simulink model "sm_cart_double_pendulum"  (R2021b)
settings: Solver=ode45  StartTime=0.0  StopTime=10  MaxStep=0.01  RelTol=1e-6  AbsTol=1e-6  EnableMultiTasking=on
undefined symbols (not defined in the file): sys_cart_dpen, X, Y, Z
libraries: sm_lib x23, nesl_utility x9, simulink x1
CloseFcn:
  | clear sys_cart_dpen
Description:
  | Inverted Double Pendulum on a Sliding Cart
  | 
  | This example shows how to model an inverted double pendulum mounted on a sliding cart using Simscape Multibody(TM). It also illustrates the use of a controller to balance the pendulum in the upright position. Make any changes to the system and click on the blue box to generate linearized model for the system before running the simulation. The control gains are computed using the linearized model. The pole placement technique is used to compute the control gains from the linearized model. The controller keeps the double pendulum vertical in the presence of a random disturbance force. See the files sm_cart_dpen_linearize.m and sm_cart_dpen_control_gains.m for details.
settings Model: Creator=The MathWorks, Inc.  LastModifiedBy=The MathWorks, Inc.
settings SolverCC: AutoScaleAbsTol=off  AlgebraicLoopSolver=TrustRegion
settings DataIOCC: LimitDataPoints=on  SaveFormat=Array  SaveOutput=off  SignalLogging=off  SaveTime=off  ReturnWorkspaceOutputs=off
settings OptimizationCC: DefaultParameterBehavior=Inlined  BufferReuse=off  ExpressionDepthLimit=2147483647  LifeSpan=inf
settings DebuggingCC: UnderspecifiedInitializationDetection=Classic  MergeDetectMultiDrivingBlocksExec=none  SolverPrmCheckMsg=warning  FcnCallInpInsideContextMsg=warning  UnconnectedInputMsg=none  AllowSymbolicDim=off  StateNameClashWarn=warning  InitInArrayFormatMsg=none  SFUnexpectedBacktrackingDiag=warning  SFNoUnconditionalDefaultTransitionDiag=warning  SFExecutionAtInitializationDiag=none  SFMachineParentedDataDiag=warning  ArithmeticOperatorsInVariantConditions=warning
settings HardwareCC: ProdBitPerPointer=32  ProdBitPerSizeT=32  ProdBitPerPtrDiffT=32  ProdLargestAtomicFloat=None  ProdIntDivRoundTo=Undefined  ProdEndianess=Unspecified  ProdWordSize=32  ProdHWDeviceType=32-bit Generic
settings ModelReferenceCC: PropagateSignalLabelsOutOfModel=off
settings SFSimCC: SimUseLocalCustomCode=off  CustomCodeUndefinedFunction=UseInterfaceOnly
settings RTWCC: RTWUseLocalCustomCode=off
settings CodeAppCC: StateflowObjectComments=on
settings GRTTargetCC: TargetLangStandard=C89/C90 (ANSI)  CombineOutputUpdateFcns=off  GRTInterface=on
settings ConfigComp: CovMetricSettings=dw  CovSaveCumulativeToWorkspaceVar=on  CovSaveSingleToWorkspaceVar=on  CovExternalEMLEnable=off  CovSFcnEnable=off
settings SimscapeCC: SimscapeNormalizeSystem=off
settings ConfigurationSet: Description=SimMechanics 2G
settings ExplorerConfigSet: InternalSimMechanicsExplorerSettings="<ExplorerConfiguration><canonicalview>default</canonicalview><TilePanel><TileInfo><Tiles Columns=\"1\" Count=\"1\" Rows=\"1\"><Column Left=\"2\" Weight=\"1\"/><Column Left=\"461\"/><Row Top=\"2\" Weight=\"1\"/><Row Top=\"419\"/><Tile Height=\"1\" Width=\"1\" X=\"0\" Y=\"0\"/></Tiles></TileInfo><SceneInfo><SceneViewer><BGColor><R>0.60000002384185791</R><G>0.60000002384185791</G><B>0.60000002384185791</B></BGColor><Camera><Position><X>0.59825210896441083</X><Y>-0.62075210985848051</Y><Z>0.77498517063566785</Z></Position><Center><X>0</X><Y>-0.022500000894069672</Y><Z>0.17673306167125702</Z></Center><Up><X>-0.40824829046386307</X><Y>0.40824829046386307</Y><Z>0.81649658092772615</Z></Up><Left>-0.2914164036512375</Left><Right>0.2914164036512375</Right><Bottom>-0.31976635158061983</Bottom><Top>0.31976635158061983</Top></Camera></SceneViewer></SceneInfo></TilePanel></ExplorerConfiguration>"

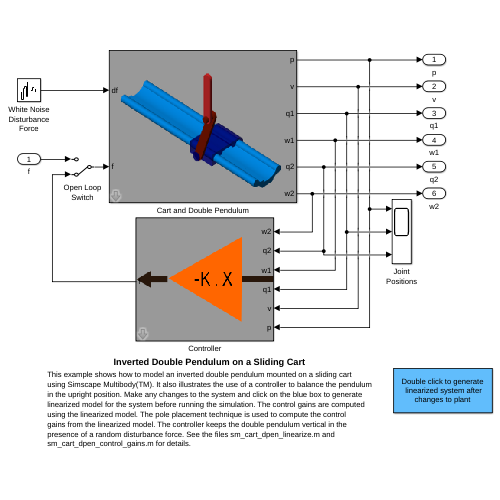
[thumbnail: Simulink's stored preview of the top-level diagram]
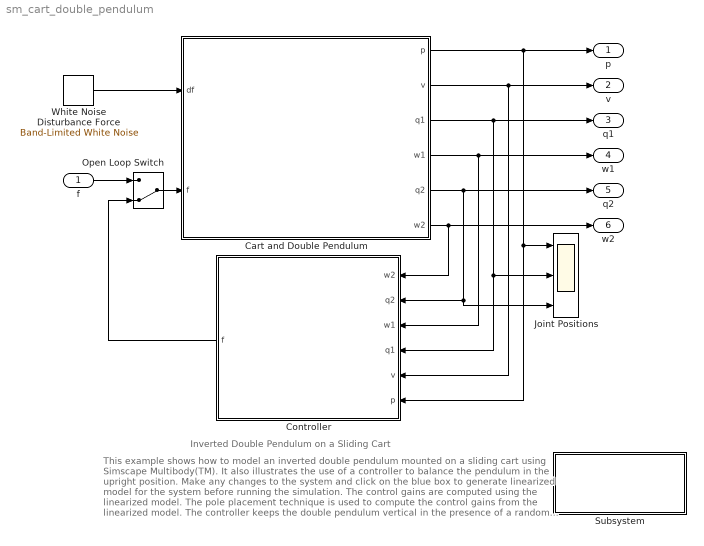
== system sm_cart_double_pendulum ==
  note: This example shows how to model an inverted double pendulum mounted on a sliding cart
      | using Simscape Multibody(TM). It also illustrates the use of a controller to balance the pendulum
      | in the upright position. Make any changes to the system and click on the blue box to generate
      | linearized model for the system before running the simulation. The control gains are computed
      | using the linearized model. The pole placement technique is used to compute the control
      | gains from the linearized model. The controller keeps the double pendulum vertical in the
      | presence of a random disturbance force. See the files sm_cart_dpen_linearize.m and
      | sm_cart_dpen_control_gains.m for details.
  note: Inverted Double Pendulum on a Sliding Cart
  f : Inport
  Cart and Double Pendulum : Subsystem  mask(Double Pendulum on a Sliding Cart){Ll=18, Lu=14, p=7, v=0, q1=-20, w1=0, q2=20, w2=0}
      mask prompts: Ll "Lower link length (cm)"; Lu "Upper link length (cm)"; p "Cart initial position (cm)"; v "Cart initial velocity (cm/s)"; q1 "Lower link initial position (deg)"; w1 "Lower link initial velocity (deg/s)"; q2 "Upper link initial position (deg)"; w2 "Upper link initial velocity (deg/s)"
      mask help:
      | Set the lengths of the pendulum links and the initial states of the joint positions and velocities in the dialog below. For other changes to the system, right click on the block and select Look Under Mask to edit the system directly.
      |
      | After any changes to the system, double click on the blue box titled "Double click to linearize system" before proceeding to simulate the model. This generates the linearized model (about the vertical upright position) of the system. The linearized system is used by the controller to compute the control gains.
      mask Display:
      | image('sm_cartdpen_full.png');
      | port_label('input',1,'df');
      | port_label('input',2,'f');
      | port_label('output',1,'p');
      | port_label('output',2,'v');
      | port_label('output',3,'q1');
      | port_label('output',4,'w1');
      | port_label('output',5,'q2');
      | port_label('output',6,'w2');
  Controller : Subsystem  mask(Controller){poles=[-11 -10 -10 -10 -10 -10], sys=sys_cart_dpen}
      mask prompts: poles "Closed Loop Desired Pole Locations (1x6 vector)"; sys "Linearized system model"
      mask help: The controller gains are computed using the Ackermann's formula for pole placement. Specify the desired closed loop pole locations (1x6 vector) in the dialog below.
      mask init:
      | if isempty(sys)
      |     K_pp = [70.5210   41.6715 -110.3868  -24.2497 -218.6747  -18.6261];
      |     Cinv = diag([1/100 1/100 1/57.2958 1/57.2958 1/57.2958 1/57.2958]);
      | else
      |     K_pp = sm_cart_dpen_control_gains(sys,poles);
      |     Cinv = inv(sys.C);
      | end
      mask Display:
      | image('sm_cartdpen_ctrl.png');
      | port_label('output',1,'f');
      | port_label('input',6,'p');
      | port_label('input',5,'v');
      | port_label('input',4,'q1');
      | port_label('input',3,'w1');
      | port_label('input',2,'q2');
      | port_label('input',1,'w2');
  Joint Positions : Scope  NumInputPorts=3
  Open Loop Switch : ManualSwitch  CurrentSetting=0
  Subsystem : Subsystem
      settings: OpenFcn=sm_cart_dpen_linearize();
      mask Display: disp('Double click to generate\n linearized system after\nchanges to plant');
  White Noise Disturbance Force : simulink/Sources/Band-Limited White Noise  Cov=1e-4  Ts=0.1  seed=[23341]
  p : Outport  VectorParamsAs1DForOutWhenUnconnected=off
  v : Outport  Port=2  VectorParamsAs1DForOutWhenUnconnected=off
  q1 : Outport  Port=3  VectorParamsAs1DForOutWhenUnconnected=off
  w1 : Outport  Port=4  VectorParamsAs1DForOutWhenUnconnected=off
  q2 : Outport  Port=5  VectorParamsAs1DForOutWhenUnconnected=off
  w2 : Outport  Port=6  VectorParamsAs1DForOutWhenUnconnected=off
  wires:
  f/1 -> Open Loop Switch/1
  Open Loop Switch/1 -> Cart and Double Pendulum/2(f)
  Cart and Double Pendulum/6(w2) -> Controller/1(w2), w2/1
  Cart and Double Pendulum/5(q2) -> q2/1, Joint Positions/3, Controller/2(q2)
  Cart and Double Pendulum/4(w1) -> Controller/3(w1), w1/1
  Cart and Double Pendulum/3(q1) -> q1/1, Controller/4(q1), Joint Positions/2
  Cart and Double Pendulum/2(v) -> Controller/5(v), v/1
  Cart and Double Pendulum/1(p) -> p/1, Controller/6(p), Joint Positions/1
  Controller/1(f) -> Open Loop Switch/2
  White Noise Disturbance Force/1 -> Cart and Double Pendulum/1(df)

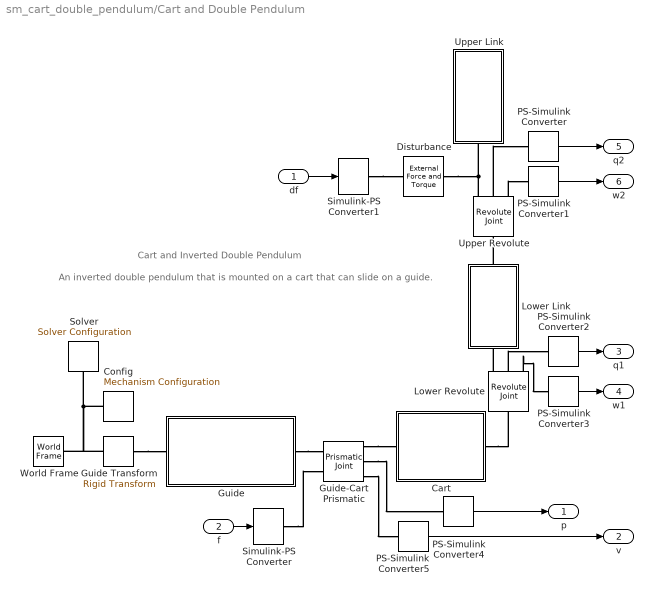
== system sm_cart_double_pendulum/Cart and Double Pendulum ==
  note: An inverted double pendulum that is mounted on a cart that can slide on a guide.
  note: Cart and Inverted Double Pendulum
  df : Inport
  f : Inport  Port=2
  Cart : Subsystem  mask(Cart){W=10, Rs=1.2, Rm=2, L=10, Rp=1, Lp=2, Rf=1.5, Tf=0.25, rho=2700, Op=0.6}
      mask prompts: W "Cart width (cm)"; Rs "Slider cavity radius (cm)"; Rm "Radius of curvature of outer surface (cm)"; L "Cart length (cm)"; Rp "Peg radius (cm)"; Lp "Peg length (cm)"; Rf "Peg Flange radius (cm)"; Tf "Peg flange thickness (cm)"; rho "Density"; Op "Opacity (cm)"
      mask help: Cart slides on a guide structure and has a peg to hang the double pendulum
      mask init:
      | theta = (180:-1:-90)*pi/180;
      | cx = W/2; cy = 0;
      | x1 = cx + 1.1*Rs*cos(theta');
      | y1 = cy + 1.1*Rs*sin(theta');
      | 
      | theta = (-90:1:90)*pi/180;
      | cx = W/2; cy = 0;
      | x2 = cx + Rm*cos(theta');
      | y2 = cy + Rm*sin(theta');
      | 
      | x3 = [-(W/2+Rm); -(W/2+Rm); -W/2];
      | y3 = [Rm; -Rm; -Rm];
      | 
      | x = [x1; x2; x3];
      | y = [y1; y2; y3];
      | 
      | x = [x ; -flipud(x1); -W/4; -W/5; W/5; W/4];
      | y = [y ;  flipud(y1); 0; Rm/2; Rm/2; 0];
      | 
      | cross_section = [x y];
      mask Display: image('sm_cartdpen_cart.png')
  Config : sm_lib/Utilities/Mechanism Configuration  UniformGravity=Constant  GravityVector=[0 0 -9.81]  GravityUnits=m/s^2  LinearizationDelta=0.001  JointModeTransitionNonlinearIterations=2
  Disturbance : sm_lib/Forces and Torques/External Force and Torque  ForceResolutionFrame=World  EnableForceX=on  EnableForceY=off  EnableForceZ=off  EnableForce=off  TorqueResolutionFrame=AttachedFrame  EnableTorqueX=off  EnableTorqueY=off  EnableTorqueZ=off  EnableTorque=off
  Guide : Subsystem  mask(Guide){W=10, Rs=1.2, Rm=3, Rl=6, L=60, Rg=1.5, rho=2700}
      mask prompts: W "Guide width (cm)"; Rs "Slider rod radius (cm)"; Rm "Underside curvature radius (cm)"; Rl "Upperside curvature radius (cm)"; L "Guide length (cm)"; Rg "Center to rack distance (cm)"; rho "Density"
      mask help: Guide structure on which the card slides
      mask init:
      | phi = asin((W/2-Rs)/Rl);
      | theta = (-phi*3/4:(-1/180):-phi) - pi/2;
      | cx = 0; cy = Rm-Rm*sin(25*pi/180)  + Rl*cos(phi) + Rs;
      | 
      | x2 = cx + Rl*cos(theta');
      | y2 = cy + Rl*sin(theta');
      | 
      | theta = (phi:(-1/180):0.01) - pi/2;
      | x5 = cx + Rl*cos(theta');
      | y5 = cy + Rl*sin(theta');
      | 
      | x1 = [0; -Rg; -Rg];
      | y1 = [cy-Rl; cy-Rl; y2(1)];
      | 
      | theta = (0:1:270)*pi/180;
      | cx = -W/2; cy = Rm-Rm*sin(25*pi/180)+Rs;
      | 
      | x3 = cx + Rs*cos(theta');
      | y3 = cy + Rs*sin(theta');
      | 
      | theta = (89:-1:25)*pi/180;
      | cx = -W/2; cy = -Rm*sin(25*pi/180);
      | 
      | x4 = cx + Rm*cos(theta');
      | y4 = cy + Rm*sin(theta');
      | 
      | x = [x1; x2; x3; x4; -flipud([x3;x4]); x5];
      | y = [y1; y2; y3; y4;  flipud([y3;y4]); y5];
      | 
      | cross_section = [x y];
      mask Display: image('sm_cartdpen_guide.png')
  Guide Transform : sm_lib/Frames and Transforms/Rigid Transform  TranslationMethod=None  TranslationStandardOffset=0  TranslationLengthUnit=m  TranslationStandardAxis=+Z  TranslationCartesianOffset=[0 0 0]  TranslationROffset=0  TranslationROffsetUnits=m  TranslationZOffset=0  TranslationZOffsetUnits=m  TranslationThetaOffset=0  TranslationThetaOffsetUnits=deg  RotationMethod=AlignedAxes  RotationAngleUnits=deg  RotationStandardAxis=+Z  RotationAngle=0  RotationArbitraryAxis=[0 0 1]  FollAlignAxisA=+Z  BaseAlignAxisA=+X  FollAlignAxisB=+X  BaseAlignAxisB=+Y  RotationSequenceAxes=FollowerAxes  RotationSequence=XYX  RotationSequenceAngles=[0 0 0]  RotationSequenceAnglesUnits=deg  RotationMatrix=[1 0 0; 0 1 0; 0 0 1]
  Guide-Cart Prismatic : sm_lib/Joints/Prismatic Joint  JointMode=Normal  SenseConstraintForce=off  SenseConstraintForceX=off  SenseConstraintForceY=off  SenseConstraintForceZ=off  SenseConstraintTorque=off  SenseConstraintTorqueX=off  SenseConstraintTorqueY=off  SenseConstraintTorqueZ=off  SenseTotalForce=off  SenseTotalForceX=off  SenseTotalForceY=off  SenseTotalForceZ=off  SenseTotalTorque=off  SenseTotalTorqueX=off  SenseTotalTorqueY=off  SenseTotalTorqueZ=off  CompositeWrenchDir=FollowerOnBase  CompositeWrenchFrame=BaseFrame  EquilibriumPosition=0  EquilibriumPositionUnits=m  SpringStiffness=0  SpringStiffnessUnits=N/m  DampingCoefficient=0  DampingCoefficientUnits=N/(m/s)  TorqueActuationMode=InputTorque  MotionActuationMode=ComputedMotion  SensePosition=on  SenseVelocity=on  SenseAcceleration=off  SenseTorqueForce=off  SenseLowerLimitTorqueForce=off  SenseUpperLimitTorqueForce=off  LowerLimitSpecify=off  LowerLimitBound=-1  LowerLimitBoundUnits=m  LowerLimitStiffness=1e6  LowerLimitStiffnessUnits=N/m  LowerLimitDamping=1e3  LowerLimitDampingUnits=N/(m/s)  LowerLimitTransitionRegionWidth=1e-4  LowerLimitTransitionRegionWidthUnits=m  UpperLimitSpecify=off  UpperLimitBound=1  UpperLimitBoundUnits=m  UpperLimitStiffness=1e6  UpperLimitStiffnessUnits=N/m  UpperLimitDamping=1e3  UpperLimitDampingUnits=N/(m/s)  UpperLimitTransitionRegionWidth=1e-4  UpperLimitTransitionRegionWidthUnits=m  PositionTargetSpecify=on  PositionTargetPriority=High  PositionTargetValue=p  PositionTargetValueUnits=cm  VelocityTargetSpecify=on  VelocityTargetPriority=High  VelocityTargetValue=v  VelocityTargetValueUnits=cm/s
  Lower Link : Subsystem  mask(Upper Link){rho=2700, L=Ll, W=3, T=1, r=1, Lp=3, clr=[0.6 0.1 0]}
      mask prompts: rho "Link density (kg/m^3):"; L "Link length (cm):"; W "Link width (cm):"; T "Link thickness (cm):"; r "Peg/Hole radius (cm):"; Lp "Peg length (cm):"; clr "Link color:"
      mask help: Upper link of the double pendulum mechanisn
      mask init:
      | % Main link cross-section
      | top_xsec = [L/2 W/2; -L/2 W/2];
      | theta = (90:-1:-90)*pi/180;
      | semi_hole_xsec = [-L/2+r*cos(theta') r*sin(theta')];
      | bottom_xsec = [-L/2 -W/2; L/2 -W/2];
      | theta = (-89:1:89)*pi/180;
      | right_end_xsec = [L/2+(W/2)*cos(theta') (W/2)*sin(theta')];
      | link_x_section = [ top_xsec; semi_hole_xsec; bottom_xsec; right_end_xsec];
      | 
      | % Left end cap cross-section
      | theta = (90:1:270)*pi/180;
      | outer_xsec = [(W/2)*cos(theta') (W/2)*sin(theta')];
      | theta = (270:-1:90)*pi/180;
      | inner_xsec = [r*cos(theta') r*sin(theta')];
      | left_end_x_section = [outer_xsec; inner_xsec];
      mask Display: image('sm_cartdpen_lowerlink.png');
  Lower Revolute : sm_lib/Joints/Revolute Joint  JointMode=Normal  SenseConstraintForce=off  SenseConstraintForceX=off  SenseConstraintForceY=off  SenseConstraintForceZ=off  SenseConstraintTorque=off  SenseConstraintTorqueX=off  SenseConstraintTorqueY=off  SenseConstraintTorqueZ=off  SenseTotalForce=off  SenseTotalForceX=off  SenseTotalForceY=off  SenseTotalForceZ=off  SenseTotalTorque=off  SenseTotalTorqueX=off  SenseTotalTorqueY=off  SenseTotalTorqueZ=off  CompositeWrenchDir=FollowerOnBase  CompositeWrenchFrame=BaseFrame  EquilibriumPosition=0  EquilibriumPositionUnits=rad  SpringStiffness=0  SpringStiffnessUnits=N*m/rad  DampingCoefficient=0  DampingCoefficientUnits=N*m/(rad/s)  TorqueActuationMode=NoTorque  MotionActuationMode=ComputedMotion  SensePosition=on  SenseVelocity=on  SenseAcceleration=off  SenseTorqueForce=off  SenseLowerLimitTorqueForce=off  SenseUpperLimitTorqueForce=off  LowerLimitSpecify=off  LowerLimitBound=-90  LowerLimitBoundUnits=deg  LowerLimitStiffness=1e4  LowerLimitStiffnessUnits=N*m/deg  LowerLimitDamping=10  LowerLimitDampingUnits=N*m/(deg/s)  LowerLimitTransitionRegionWidth=0.1  LowerLimitTransitionRegionWidthUnits=deg  UpperLimitSpecify=off  UpperLimitBound=90  UpperLimitBoundUnits=deg  UpperLimitStiffness=1e4  UpperLimitStiffnessUnits=N*m/deg  UpperLimitDamping=10  UpperLimitDampingUnits=N*m/(deg/s)  UpperLimitTransitionRegionWidth=0.1  UpperLimitTransitionRegionWidthUnits=deg  PositionTargetSpecify=on  PositionTargetPriority=High  PositionTargetValue=q1  PositionTargetValueUnits=deg  VelocityTargetSpecify=on  VelocityTargetPriority=Low  VelocityTargetValue=w1  VelocityTargetValueUnits=deg/s
  PS-Simulink Converter : nesl_utility/PS-Simulink Converter  PhysicalDomain=network_engine_domain  SubClassName=ps_output  LeftPortType=input  RightPortType=output  PseudoPeriodic=off  Frequencies=[]  Unit=deg  AffineConversion=off
      settings: SourceProductBaseCode=PW,SS
  PS-Simulink Converter1 : nesl_utility/PS-Simulink Converter  PhysicalDomain=network_engine_domain  SubClassName=ps_output  LeftPortType=input  RightPortType=output  PseudoPeriodic=off  Frequencies=[]  Unit=deg/s  AffineConversion=off
      settings: SourceProductBaseCode=PW,SS
  PS-Simulink Converter2 : nesl_utility/PS-Simulink Converter  PhysicalDomain=network_engine_domain  SubClassName=ps_output  LeftPortType=input  RightPortType=output  PseudoPeriodic=off  Frequencies=[]  Unit=deg  AffineConversion=off
      settings: SourceProductBaseCode=PW,SS
  PS-Simulink Converter3 : nesl_utility/PS-Simulink Converter  PhysicalDomain=network_engine_domain  SubClassName=ps_output  LeftPortType=input  RightPortType=output  PseudoPeriodic=off  Frequencies=[]  Unit=deg/s  AffineConversion=off
      settings: SourceProductBaseCode=PW,SS
  PS-Simulink Converter4 : nesl_utility/PS-Simulink Converter  PhysicalDomain=network_engine_domain  SubClassName=ps_output  LeftPortType=input  RightPortType=output  PseudoPeriodic=off  Frequencies=[]  Unit=cm  AffineConversion=off
      settings: SourceProductBaseCode=PW,SS
  PS-Simulink Converter5 : nesl_utility/PS-Simulink Converter  PhysicalDomain=network_engine_domain  SubClassName=ps_output  LeftPortType=input  RightPortType=output  PseudoPeriodic=off  Frequencies=[]  Unit=cm/s  AffineConversion=off
      settings: SourceProductBaseCode=PW,SS
  Simulink-PS Converter : nesl_utility/Simulink-PS Converter  PhysicalDomain=network_engine_domain  SubClassName=ps_input  LeftPortType=input  RightPortType=output  PseudoPeriodic=off  Frequencies=[]  NoiseDistribution=none  NoiseParameters=[]  Unit=N  AffineConversion=off  FilteringAndDerivatives=zero  SimscapeFilterOrder=1  InputFilterTimeConstant=.001  UdotUserProvided=1
      settings: SourceProductBaseCode=PW,SS
  Simulink-PS Converter1 : nesl_utility/Simulink-PS Converter  PhysicalDomain=network_engine_domain  SubClassName=ps_input  LeftPortType=input  RightPortType=output  PseudoPeriodic=off  Frequencies=[]  NoiseDistribution=none  NoiseParameters=[]  Unit=N  AffineConversion=off  FilteringAndDerivatives=zero  SimscapeFilterOrder=1  InputFilterTimeConstant=.001  UdotUserProvided=1
      settings: SourceProductBaseCode=PW,SS
  Solver : nesl_utility/Solver Configuration  PhysicalDomain=network_engine_domain  SubClassName=solver  LeftPortType=input  RightPortType=generic  Tones=[]  Harmonics=[]  SimulateNoise=off  Profile=off  UseLocalSampling=off  EnableSwitchedLinearOptims=on  FrequencyDomain=off  UseCCode=off  RelTol=0.001  AbsTol=1e-06  MinStep=1e-09  ToWorkspace=off  RevertToSquareIcSolve=off  NumHomotopyIterations=100  PhasorMode=off  PhasorModeNumHarmonics=1  DoDC=off  ResidualTolerance=1e-9  UseLocalSolver=off  LocalSolverChoice=NE_BACKWARD_EULER_ADVANCER  LocalSolverSampleTime=.001  DoFixedCost=off  MaxNonlinIter=3  MaxModeIter=2  ComputeImpulses=off  ImpulseIterations=2  LinearAlgebra=Sparse  EquationFormulation=NE_TIME_EF  DelaysMemoryBudget=1024  AutomaticFiltering=on  FilteringTimeConstant=0.001  PartitionStorageMethod=AS_NEEDED  PartitionMemoryBudget=1024  PartitionMethod=FAST
      settings: SourceProductBaseCode=PW,SS
  Upper Link : Subsystem  mask(Upper Link){rho=2700, L=Lu, W=3, T=1, r=1, clr=[1 0.2 0.2]}
      mask prompts: rho "Link density (kg/m^3):"; L "Link length (cm):"; W "Link width (cm):"; T "Link thickness (cm):"; r "Hole radius (cm):"; clr "Link color:"
      mask help: Upper link of the double pendulum mechanisn
      mask init:
      | % Main link cross-section
      | top_xsec = [L/2 W/2; -L/2 W/2];
      | theta = (90:-1:-90)*pi/180;
      | semi_hole_xsec = [-L/2+r*cos(theta') r*sin(theta')];
      | bottom_xsec = [-L/2 -W/2; L/2 -W/2];
      | theta = (-89:1:89)*pi/180;
      | right_end_xsec = [L/2+(W/2)*cos(theta') (W/2)*sin(theta')];
      | link_x_section = [ top_xsec; semi_hole_xsec; bottom_xsec; right_end_xsec];
      | 
      | % Left end cap cross-section
      | theta = (90:1:270)*pi/180;
      | outer_xsec = [(W/2)*cos(theta') (W/2)*sin(theta')];
      | theta = (270:-1:90)*pi/180;
      | inner_xsec = [r*cos(theta') r*sin(theta')];
      | left_end_x_section = [outer_xsec; inner_xsec];
      mask Display: image('sm_cartdpen_upperlink.png');
  Upper Revolute : sm_lib/Joints/Revolute Joint  JointMode=Normal  SenseConstraintForce=off  SenseConstraintForceX=off  SenseConstraintForceY=off  SenseConstraintForceZ=off  SenseConstraintTorque=off  SenseConstraintTorqueX=off  SenseConstraintTorqueY=off  SenseConstraintTorqueZ=off  SenseTotalForce=off  SenseTotalForceX=off  SenseTotalForceY=off  SenseTotalForceZ=off  SenseTotalTorque=off  SenseTotalTorqueX=off  SenseTotalTorqueY=off  SenseTotalTorqueZ=off  CompositeWrenchDir=FollowerOnBase  CompositeWrenchFrame=BaseFrame  EquilibriumPosition=0  EquilibriumPositionUnits=rad  SpringStiffness=0  SpringStiffnessUnits=N*m/rad  DampingCoefficient=0  DampingCoefficientUnits=N*m/(rad/s)  TorqueActuationMode=NoTorque  MotionActuationMode=ComputedMotion  SensePosition=on  SenseVelocity=on  SenseAcceleration=off  SenseTorqueForce=off  SenseLowerLimitTorqueForce=off  SenseUpperLimitTorqueForce=off  LowerLimitSpecify=off  LowerLimitBound=-90  LowerLimitBoundUnits=deg  LowerLimitStiffness=1e4  LowerLimitStiffnessUnits=N*m/deg  LowerLimitDamping=10  LowerLimitDampingUnits=N*m/(deg/s)  LowerLimitTransitionRegionWidth=0.1  LowerLimitTransitionRegionWidthUnits=deg  UpperLimitSpecify=off  UpperLimitBound=90  UpperLimitBoundUnits=deg  UpperLimitStiffness=1e4  UpperLimitStiffnessUnits=N*m/deg  UpperLimitDamping=10  UpperLimitDampingUnits=N*m/(deg/s)  UpperLimitTransitionRegionWidth=0.1  UpperLimitTransitionRegionWidthUnits=deg  PositionTargetSpecify=on  PositionTargetPriority=High  PositionTargetValue=q2  PositionTargetValueUnits=deg  VelocityTargetSpecify=on  VelocityTargetPriority=Low  VelocityTargetValue=w2  VelocityTargetValueUnits=deg/s
  World Frame : sm_lib/Frames and Transforms/World Frame
  p : Outport  VectorParamsAs1DForOutWhenUnconnected=off
  v : Outport  Port=2  VectorParamsAs1DForOutWhenUnconnected=off
  q1 : Outport  Port=3  VectorParamsAs1DForOutWhenUnconnected=off
  w1 : Outport  Port=4  VectorParamsAs1DForOutWhenUnconnected=off
  q2 : Outport  Port=5  VectorParamsAs1DForOutWhenUnconnected=off
  w2 : Outport  Port=6  VectorParamsAs1DForOutWhenUnconnected=off
  wires:
  PS-Simulink Converter2/1 -> q1/1
  f/1 -> Simulink-PS Converter/1
  PS-Simulink Converter/1 -> q2/1
  PS-Simulink Converter1/1 -> w2/1
  PS-Simulink Converter3/1 -> w1/1
  PS-Simulink Converter4/1 -> p/1
  PS-Simulink Converter5/1 -> v/1
  df/1 -> Simulink-PS Converter1/1
  connections:
  Guide-Cart Prismatic/RConn1 -- Cart/LConn1
  Cart/RConn1 -- Lower Revolute/LConn1
  Guide Transform/RConn1 -- Guide/LConn1
  Guide/RConn1 -- Guide-Cart Prismatic/LConn1
  Simulink-PS Converter/RConn1 -- Guide-Cart Prismatic/LConn2
  Guide-Cart Prismatic/RConn2 -- PS-Simulink Converter4/LConn1
  Guide-Cart Prismatic/RConn3 -- PS-Simulink Converter5/LConn1
  Lower Revolute/RConn1 -- Lower Link/LConn1
  Lower Link/RConn1 -- Upper Revolute/LConn1
  Lower Revolute/RConn2 -- PS-Simulink Converter2/LConn1
  Lower Revolute/RConn3 -- PS-Simulink Converter3/LConn1
  Upper Revolute/RConn2 -- PS-Simulink Converter/LConn1
  Upper Revolute/RConn3 -- PS-Simulink Converter1/LConn1
  Simulink-PS Converter1/RConn1 -- Disturbance/LConn1
  Guide Transform/LConn1 -- World Frame/RConn1 -- Solver/RConn1 -- Config/RConn1
  Upper Revolute/RConn1 -- Upper Link/LConn1 -- Disturbance/RConn1

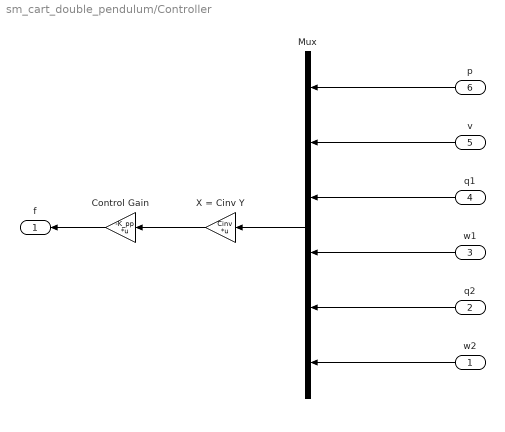
== system sm_cart_double_pendulum/Controller ==
  w2 : Inport
  q2 : Inport  Port=2
  w1 : Inport  Port=3
  q1 : Inport  Port=4
  v : Inport  Port=5
  p : Inport  Port=6
  Control Gain : Gain  Gain=-K_pp  Multiplication=Matrix(K*u)
  Mux : Mux  Inputs=6
  X = Cinv Y : Gain  Gain=Cinv  Multiplication=Matrix(K*u)
  f : Outport  VectorParamsAs1DForOutWhenUnconnected=off
  wires:
  Control Gain/1 -> f/1
  w2/1 -> Mux/6
  p/1 -> Mux/1
  q2/1 -> Mux/5
  v/1 -> Mux/2
  q1/1 -> Mux/3
  w1/1 -> Mux/4
  Mux/1 -> X = Cinv Y/1
  X = Cinv Y/1 -> Control Gain/1

== system sm_cart_double_pendulum/Subsystem ==

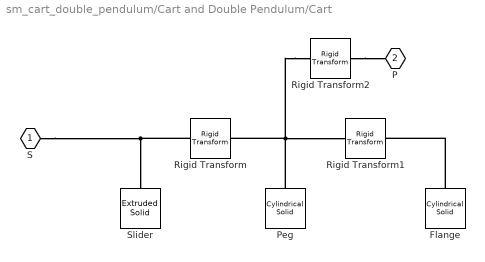
== system sm_cart_double_pendulum/Cart and Double Pendulum/Cart ==
  Flange : sm_lib/Body Elements/Cylindrical Solid  GraphicAmbientColor=[0.5 0.0 0.0 1.0]  BasedOnType=Density  CenterOfMass=[0 0 0]  CenterOfMassUnits=m  GraphicDiffuseColor=[0.0 0.0 0.6]  CylinderLength=Tf  CylinderLengthUnits=cm  CylinderRadius=Rf  CylinderRadiusUnits=cm  Density=rho  DensityUnits=kg/(m^3)  DoExposeReferenceFrame=on  GraphicEmissiveColor=[0.0 0.0 0.0 1.0]  ExportEntireGeometry=off  SerializedFrames=<Frames/>  MarkerShape=Sphere  MarkerSize=10  GraphicType=FromGeometry  InertiaType=CalculateFromGeometry  Mass=1  MassUnits=kg  MomentsOfInertia=[1 1 1]  MomentsOfInertiaUnits=kg*m^2  GraphicOpacity=Op  ProductsOfInertia=[0 0 0]  ProductsOfInertiaUnits=kg*m^2  GraphicShininess=75  GraphicSpecularColor=[0.5 0.5 0.5 1.0]  GraphicVisPropType=SimpleVisualProperties
  Peg : sm_lib/Body Elements/Cylindrical Solid  GraphicAmbientColor=[0.5 0.0 0.0 1.0]  BasedOnType=Density  CenterOfMass=[0 0 0]  CenterOfMassUnits=m  GraphicDiffuseColor=[0.0 0.0 0.6]  CylinderLength=Lp  CylinderLengthUnits=cm  CylinderRadius=Rp  CylinderRadiusUnits=cm  Density=rho  DensityUnits=kg/(m^3)  DoExposeReferenceFrame=on  GraphicEmissiveColor=[0.0 0.0 0.0 1.0]  ExportEntireGeometry=off  SerializedFrames=<Frames/>  MarkerShape=Sphere  MarkerSize=10  GraphicType=FromGeometry  InertiaType=CalculateFromGeometry  Mass=1  MassUnits=kg  MomentsOfInertia=[1 1 1]  MomentsOfInertiaUnits=kg*m^2  GraphicOpacity=Op  ProductsOfInertia=[0 0 0]  ProductsOfInertiaUnits=kg*m^2  GraphicShininess=75  GraphicSpecularColor=[0.5 0.5 0.5 1.0]  GraphicVisPropType=SimpleVisualProperties
  Rigid Transform : sm_lib/Frames and Transforms/Rigid Transform  TranslationMethod=StandardAxis  TranslationStandardOffset=W/2 + Rm + Lp/2  TranslationLengthUnit=cm  TranslationStandardAxis=-X  TranslationCartesianOffset=[0 0 0]  TranslationROffset=0  TranslationROffsetUnits=m  TranslationZOffset=0  TranslationZOffsetUnits=m  TranslationThetaOffset=0  TranslationThetaOffsetUnits=deg  RotationMethod=AlignedAxes  RotationAngleUnits=deg  RotationStandardAxis=+Z  RotationAngle=0  RotationArbitraryAxis=[0 0 1]  FollAlignAxisA=+Z  BaseAlignAxisA=-X  FollAlignAxisB=+X  BaseAlignAxisB=+Z  RotationSequenceAxes=FollowerAxes  RotationSequence=XYX  RotationSequenceAngles=[0 0 0]  RotationSequenceAnglesUnits=deg  RotationMatrix=[1 0 0; 0 1 0; 0 0 1]
  Rigid Transform1 : sm_lib/Frames and Transforms/Rigid Transform  TranslationMethod=StandardAxis  TranslationStandardOffset=Lp/2 + Tf/2  TranslationLengthUnit=cm  TranslationStandardAxis=+Z  TranslationCartesianOffset=[0 0 0]  TranslationROffset=0  TranslationROffsetUnits=m  TranslationZOffset=0  TranslationZOffsetUnits=m  TranslationThetaOffset=0  TranslationThetaOffsetUnits=deg  RotationMethod=None  RotationAngleUnits=deg  RotationStandardAxis=+Z  RotationAngle=0  RotationArbitraryAxis=[0 0 1]  FollAlignAxisA=+Z  BaseAlignAxisA=+X  FollAlignAxisB=+X  BaseAlignAxisB=-Z  RotationSequenceAxes=FollowerAxes  RotationSequence=XYX  RotationSequenceAngles=[0 0 0]  RotationSequenceAnglesUnits=deg  RotationMatrix=[1 0 0; 0 1 0; 0 0 1]
  Rigid Transform2 : sm_lib/Frames and Transforms/Rigid Transform  TranslationMethod=None  TranslationStandardOffset=0  TranslationLengthUnit=cm  TranslationStandardAxis=+Z  TranslationCartesianOffset=[0 0 0]  TranslationROffset=0  TranslationROffsetUnits=m  TranslationZOffset=0  TranslationZOffsetUnits=m  TranslationThetaOffset=0  TranslationThetaOffsetUnits=deg  RotationMethod=StandardAxis  RotationAngleUnits=deg  RotationStandardAxis=+Z  RotationAngle=90  RotationArbitraryAxis=[0 0 1]  FollAlignAxisA=+Z  BaseAlignAxisA=+X  FollAlignAxisB=+X  BaseAlignAxisB=-Z  RotationSequenceAxes=FollowerAxes  RotationSequence=XYX  RotationSequenceAngles=[0 0 0]  RotationSequenceAnglesUnits=deg  RotationMatrix=[1 0 0; 0 1 0; 0 0 1]
  Slider : sm_lib/Body Elements/Extruded Solid  GraphicAmbientColor=[0.5 0.0 0.0 1.0]  BasedOnType=Density  CenterOfMass=[0 0 0]  CenterOfMassUnits=m  GraphicDiffuseColor=[0.0 0.0 0.6]  ExportConvexHullGeometry=off  ExtrusionCrossSection=cross_section  ExtrusionCrossSectionUnits=cm  Density=rho  DensityUnits=kg/(m^3)  DoExposeReferenceFrame=on  GraphicEmissiveColor=[0.0 0.0 0.0 1.0]  ExportEntireGeometry=off  ExtrusionLength=L  ExtrusionLengthUnits=cm  ExtrusionType=General  SerializedFrames=<Frames/>  MarkerShape=Sphere  MarkerSize=10  GraphicType=FromGeometry  InertiaType=CalculateFromGeometry  Mass=1  MassUnits=kg  MomentsOfInertia=[1 1 1]  MomentsOfInertiaUnits=kg*m^2  PolygonNumSides=3  GraphicOpacity=Op  PolygonOuterRadius=1  PolygonOuterRadiusUnits=m  ProductsOfInertia=[0 0 0]  ProductsOfInertiaUnits=kg*m^2  GraphicShininess=75  GraphicSpecularColor=[0.5 0.5 0.5 1.0]  GraphicVisPropType=SimpleVisualProperties
  S : PMIOPort  Side=Left
  P : PMIOPort  Port=2  Side=Right
  connections:
  Rigid Transform2/RConn1 -- P/RConn1
  Rigid Transform2/LConn1 -- Peg/RConn1 -- Rigid Transform/RConn1 -- Rigid Transform1/LConn1
  S/RConn1 -- Rigid Transform/LConn1 -- Slider/RConn1
  Flange/RConn1 -- Rigid Transform1/RConn1

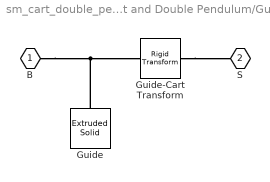
== system sm_cart_double_pendulum/Cart and Double Pendulum/Guide ==
  Guide : sm_lib/Body Elements/Extruded Solid  GraphicAmbientColor=[0.5 0.0 0.0 1.0]  BasedOnType=Density  CenterOfMass=[0 0 0]  CenterOfMassUnits=m  GraphicDiffuseColor=[0.0 0.6 1.0]  ExportConvexHullGeometry=off  ExtrusionCrossSection=cross_section  ExtrusionCrossSectionUnits=cm  Density=rho  DensityUnits=kg/(m^3)  DoExposeReferenceFrame=on  GraphicEmissiveColor=[0.0 0.0 0.0 1.0]  ExportEntireGeometry=off  ExtrusionLength=L  ExtrusionLengthUnits=cm  ExtrusionType=General  SerializedFrames=<Frames/>  MarkerShape=Sphere  MarkerSize=10  GraphicType=FromGeometry  InertiaType=CalculateFromGeometry  Mass=1  MassUnits=kg  MomentsOfInertia=[1 1 1]  MomentsOfInertiaUnits=kg*m^2  PolygonNumSides=3  GraphicOpacity=1.0  PolygonOuterRadius=1  PolygonOuterRadiusUnits=m  ProductsOfInertia=[0 0 0]  ProductsOfInertiaUnits=kg*m^2  GraphicShininess=75  GraphicSpecularColor=[0.5 0.5 0.5 1.0]  GraphicVisPropType=SimpleVisualProperties
  Guide-Cart Transform : sm_lib/Frames and Transforms/Rigid Transform  TranslationMethod=StandardAxis  TranslationStandardOffset=Rm-Rm*sin(25*pi/180)+Rs  TranslationLengthUnit=cm  TranslationStandardAxis=+Y  TranslationCartesianOffset=[0 0 0]  TranslationROffset=0  TranslationROffsetUnits=m  TranslationZOffset=0  TranslationZOffsetUnits=m  TranslationThetaOffset=0  TranslationThetaOffsetUnits=deg  RotationMethod=None  RotationAngleUnits=deg  RotationStandardAxis=+Z  RotationAngle=0  RotationArbitraryAxis=[0 0 1]  FollAlignAxisA=+Z  BaseAlignAxisA=-Z  FollAlignAxisB=+X  BaseAlignAxisB=-X  RotationSequenceAxes=FollowerAxes  RotationSequence=XYX  RotationSequenceAngles=[0 0 0]  RotationSequenceAnglesUnits=deg  RotationMatrix=[1 0 0; 0 1 0; 0 0 1]
  B : PMIOPort  Side=Left
  S : PMIOPort  Port=2  Side=Right
  connections:
  B/RConn1 -- Guide/RConn1 -- Guide-Cart Transform/LConn1
  Guide-Cart Transform/RConn1 -- S/RConn1

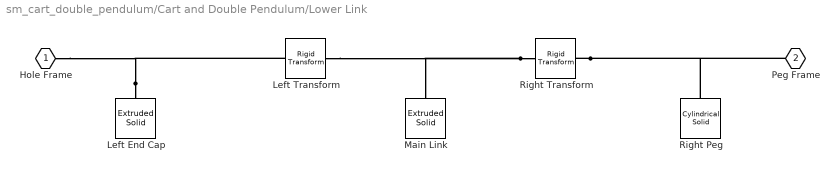
== system sm_cart_double_pendulum/Cart and Double Pendulum/Lower Link ==
  Left Transform : sm_lib/Frames and Transforms/Rigid Transform  TranslationMethod=StandardAxis  TranslationStandardOffset=L/2  TranslationLengthUnit=cm  TranslationStandardAxis=-X  TranslationCartesianOffset=[0 0 0]  TranslationROffset=0  TranslationROffsetUnits=m  TranslationZOffset=0  TranslationZOffsetUnits=m  TranslationThetaOffset=0  TranslationThetaOffsetUnits=deg  RotationMethod=None  RotationAngleUnits=deg  RotationStandardAxis=+Z  RotationAngle=0  RotationArbitraryAxis=[0 0 1]  FollAlignAxisA=+X  BaseAlignAxisA=+Y  FollAlignAxisB=+Y  BaseAlignAxisB=+Z  RotationSequenceAxes=FollowerAxes  RotationSequence=XYX  RotationSequenceAngles=[0 0 0]  RotationSequenceAnglesUnits=deg  RotationMatrix=[1 0 0; 0 1 0; 0 0 1]
  Left End Cap : sm_lib/Body Elements/Extruded Solid  GraphicAmbientColor=[0.5 0.5 0.5]  BasedOnType=Density  CenterOfMass=[0 0 0]  CenterOfMassUnits=m  GraphicDiffuseColor=clr  ExportConvexHullGeometry=off  ExtrusionCrossSection=left_end_x_section  ExtrusionCrossSectionUnits=cm  Density=rho  DensityUnits=kg/m^3  DoExposeReferenceFrame=on  GraphicEmissiveColor=[0.1 0.1 0.1]  ExportEntireGeometry=off  ExtrusionLength=T  ExtrusionLengthUnits=cm  ExtrusionType=General  SerializedFrames=<Frames/>  MarkerShape=Sphere  MarkerSize=1  GraphicType=FromGeometry  InertiaType=CalculateFromGeometry  Mass=1  MassUnits=kg  MomentsOfInertia=[1 1 1]  MomentsOfInertiaUnits=kg*m^2  PolygonNumSides=1  GraphicOpacity=1  PolygonOuterRadius=1  PolygonOuterRadiusUnits=m  ProductsOfInertia=[0 0 0]  ProductsOfInertiaUnits=kg*m^2  GraphicShininess=24.0  GraphicSpecularColor=[0.2 0.2 0.2]  GraphicVisPropType=SimpleVisualProperties
  Main Link : sm_lib/Body Elements/Extruded Solid  GraphicAmbientColor=[0.5 0.5 0.5]  BasedOnType=Density  CenterOfMass=[0 0 0]  CenterOfMassUnits=m  GraphicDiffuseColor=clr  ExportConvexHullGeometry=off  ExtrusionCrossSection=link_x_section  ExtrusionCrossSectionUnits=cm  Density=rho  DensityUnits=kg/m^3  DoExposeReferenceFrame=on  GraphicEmissiveColor=[0.1 0.1 0.1]  ExportEntireGeometry=off  ExtrusionLength=T  ExtrusionLengthUnits=cm  ExtrusionType=General  SerializedFrames=<Frames/>  MarkerShape=Sphere  MarkerSize=1  GraphicType=FromGeometry  InertiaType=CalculateFromGeometry  Mass=1  MassUnits=kg  MomentsOfInertia=[1 1 1]  MomentsOfInertiaUnits=kg*m^2  PolygonNumSides=1  GraphicOpacity=1  PolygonOuterRadius=1  PolygonOuterRadiusUnits=m  ProductsOfInertia=[0 0 0]  ProductsOfInertiaUnits=kg*m^2  GraphicShininess=24.0  GraphicSpecularColor=[0.2 0.2 0.2]  GraphicVisPropType=SimpleVisualProperties
  Right Peg : sm_lib/Body Elements/Cylindrical Solid  GraphicAmbientColor=[0.5 0.5 0.5]  BasedOnType=Density  CenterOfMass=[0 0 0]  CenterOfMassUnits=m  GraphicDiffuseColor=clr  CylinderLength=Lp  CylinderLengthUnits=cm  CylinderRadius=r  CylinderRadiusUnits=cm  Density=rho  DensityUnits=kg/m^3  DoExposeReferenceFrame=on  GraphicEmissiveColor=[0.1 0.1 0.1]  ExportEntireGeometry=off  SerializedFrames=<Frames/>  MarkerShape=Sphere  MarkerSize=1  GraphicType=FromGeometry  InertiaType=CalculateFromGeometry  Mass=1  MassUnits=kg  MomentsOfInertia=[1 1 1]  MomentsOfInertiaUnits=kg*m^2  GraphicOpacity=1  ProductsOfInertia=[0 0 0]  ProductsOfInertiaUnits=kg*m^2  GraphicShininess=24.0  GraphicSpecularColor=[0.2 0.2 0.2]  GraphicVisPropType=SimpleVisualProperties
  Right Transform : sm_lib/Frames and Transforms/Rigid Transform  TranslationMethod=Cartesian  TranslationStandardOffset=0  TranslationLengthUnit=cm  TranslationStandardAxis=+Z  TranslationCartesianOffset=[L/2 0 2*T]  TranslationROffset=0  TranslationROffsetUnits=m  TranslationZOffset=0  TranslationZOffsetUnits=m  TranslationThetaOffset=0  TranslationThetaOffsetUnits=deg  RotationMethod=None  RotationAngleUnits=deg  RotationStandardAxis=+Z  RotationAngle=0  RotationArbitraryAxis=[0 0 1]  FollAlignAxisA=+X  BaseAlignAxisA=+Y  FollAlignAxisB=+Y  BaseAlignAxisB=+Z  RotationSequenceAxes=FollowerAxes  RotationSequence=XYX  RotationSequenceAngles=[0 0 0]  RotationSequenceAnglesUnits=deg  RotationMatrix=[1 0 0; 0 1 0; 0 0 1]
  Hole Frame : PMIOPort  Side=Left
  Peg Frame : PMIOPort  Port=2  Side=Right
  connections:
  Right Transform/RConn1 -- Right Peg/RConn1 -- Peg Frame/RConn1
  Left End Cap/RConn1 -- Left Transform/RConn1 -- Hole Frame/RConn1
  Right Transform/LConn1 -- Main Link/RConn1 -- Left Transform/LConn1

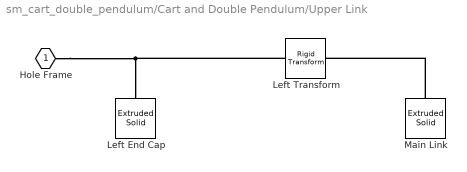
== system sm_cart_double_pendulum/Cart and Double Pendulum/Upper Link ==
  Left Transform : sm_lib/Frames and Transforms/Rigid Transform  TranslationMethod=StandardAxis  TranslationStandardOffset=L/2  TranslationLengthUnit=cm  TranslationStandardAxis=-X  TranslationCartesianOffset=[0 0 0]  TranslationROffset=0  TranslationROffsetUnits=m  TranslationZOffset=0  TranslationZOffsetUnits=m  TranslationThetaOffset=0  TranslationThetaOffsetUnits=deg  RotationMethod=None  RotationAngleUnits=deg  RotationStandardAxis=+Z  RotationAngle=0  RotationArbitraryAxis=[0 0 1]  FollAlignAxisA=+X  BaseAlignAxisA=+Y  FollAlignAxisB=+Y  BaseAlignAxisB=+Z  RotationSequenceAxes=FollowerAxes  RotationSequence=XYX  RotationSequenceAngles=[0 0 0]  RotationSequenceAnglesUnits=deg  RotationMatrix=[1 0 0; 0 1 0; 0 0 1]
  Left End Cap : sm_lib/Body Elements/Extruded Solid  GraphicAmbientColor=[0.5 0.5 0.5]  BasedOnType=Density  CenterOfMass=[0 0 0]  CenterOfMassUnits=m  GraphicDiffuseColor=clr  ExportConvexHullGeometry=off  ExtrusionCrossSection=left_end_x_section  ExtrusionCrossSectionUnits=cm  Density=rho  DensityUnits=kg/m^3  DoExposeReferenceFrame=on  GraphicEmissiveColor=[0.1 0.1 0.1]  ExportEntireGeometry=off  ExtrusionLength=T  ExtrusionLengthUnits=cm  ExtrusionType=General  SerializedFrames=<Frames/>  MarkerShape=Sphere  MarkerSize=1  GraphicType=FromGeometry  InertiaType=CalculateFromGeometry  Mass=1  MassUnits=kg  MomentsOfInertia=[1 1 1]  MomentsOfInertiaUnits=kg*m^2  PolygonNumSides=1  GraphicOpacity=1  PolygonOuterRadius=1  PolygonOuterRadiusUnits=m  ProductsOfInertia=[0 0 0]  ProductsOfInertiaUnits=kg*m^2  GraphicShininess=24.0  GraphicSpecularColor=[0.2 0.2 0.2]  GraphicVisPropType=SimpleVisualProperties
  Main Link : sm_lib/Body Elements/Extruded Solid  GraphicAmbientColor=[0.5 0.5 0.5]  BasedOnType=Density  CenterOfMass=[0 0 0]  CenterOfMassUnits=m  GraphicDiffuseColor=clr  ExportConvexHullGeometry=off  ExtrusionCrossSection=link_x_section  ExtrusionCrossSectionUnits=cm  Density=rho  DensityUnits=kg/m^3  DoExposeReferenceFrame=on  GraphicEmissiveColor=[0.1 0.1 0.1]  ExportEntireGeometry=off  ExtrusionLength=T  ExtrusionLengthUnits=cm  ExtrusionType=General  SerializedFrames=<Frames/>  MarkerShape=Sphere  MarkerSize=1  GraphicType=FromGeometry  InertiaType=CalculateFromGeometry  Mass=1  MassUnits=kg  MomentsOfInertia=[1 1 1]  MomentsOfInertiaUnits=kg*m^2  PolygonNumSides=1  GraphicOpacity=1  PolygonOuterRadius=1  PolygonOuterRadiusUnits=m  ProductsOfInertia=[0 0 0]  ProductsOfInertiaUnits=kg*m^2  GraphicShininess=24.0  GraphicSpecularColor=[0.2 0.2 0.2]  GraphicVisPropType=SimpleVisualProperties
  Hole Frame : PMIOPort  Side=Left
  connections:
  Main Link/RConn1 -- Left Transform/LConn1
  Hole Frame/RConn1 -- Left Transform/RConn1 -- Left End Cap/RConn1
